simulink model "FeedBack_Linearization"  (R2021b)
settings: Solver=VariableStepAuto  StartTime=0.0  StopTime=10.0  RelTol=1e-3
undefined symbols (not defined in the file or in its folder): Kd, Kp, q_dq_init
(part 1 of 3)
settings Model: Creator=Yafei Ou  LastModifiedBy=ouyaf

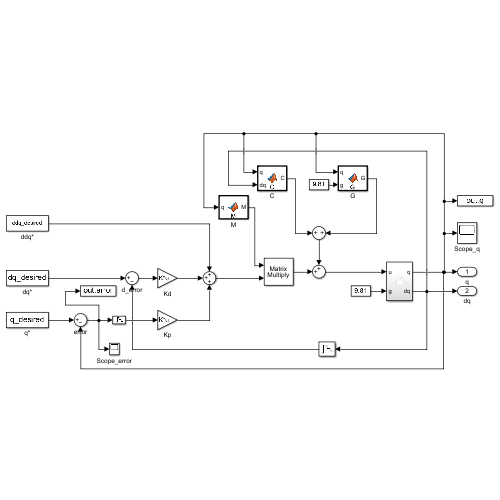
[thumbnail: Simulink's stored preview of the top-level diagram]
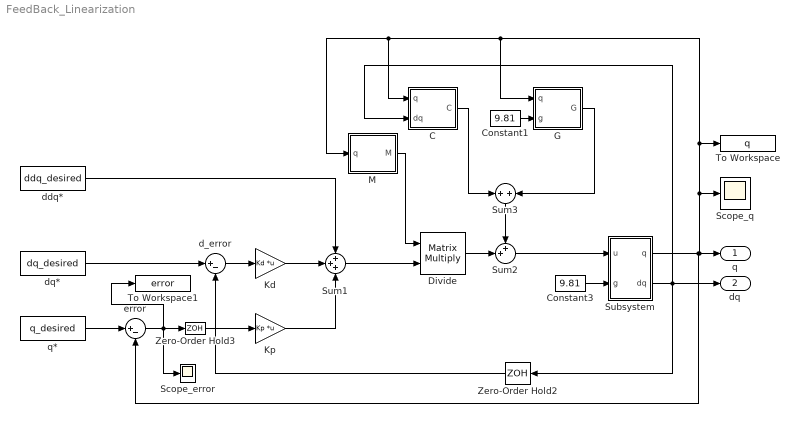
== system FeedBack_Linearization ==
  C : MATLAB Function  TreatAsAtomicUnit=on
  Constant1 : Constant  Value=9.81
  Constant3 : Constant  Value=9.81
  Divide : Product  Inputs=**  Multiplication=Matrix(*)
  G : MATLAB Function  TreatAsAtomicUnit=on
  Kd : Gain  Gain=Kd  Multiplication=Matrix(K*u)
  Kp : Gain  Gain=Kp  Multiplication=Matrix(K*u)
  M : MATLAB Function  TreatAsAtomicUnit=on
  Scope_error : Scope
  Scope_q : Scope
  Subsystem : Subsystem
  Sum1 : Sum  Inputs=+++
  Sum2 : Sum  Inputs=++|
  Sum3 : Sum  Inputs=+|+
  To Workspace : ToWorkspace  VariableName=q  SaveFormat=Timeseries  SampleTime=-1
  To Workspace1 : ToWorkspace  VariableName=error  SaveFormat=Timeseries  SampleTime=-1
  Zero-Order Hold2 : ZeroOrderHold  SampleTime=0.01
  Zero-Order Hold3 : ZeroOrderHold  SampleTime=0.01
  d_error : Sum  Inputs=|+-
  ddq* : FromWorkspace  VariableName=ddq_desired
  dq* : FromWorkspace  VariableName=dq_desired
  error : Sum  Inputs=|+-
  q* : FromWorkspace  VariableName=q_desired
  q : Outport  PortDimensions=6
  dq : Outport  Port=2
  wires:
  M/1(M) -> Divide/1
  Zero-Order Hold2/1 -> d_error/2
  C/1(C) -> Sum3/1
  Kp/1 -> Sum1/3
  Divide/1 -> Sum2/2
  Kd/1 -> Sum1/2
  dq*/1 -> d_error/1
  error/1 -> Zero-Order Hold3/1, Scope_error/1, To Workspace1/1
  Sum1/1 -> Divide/2
  Constant1/1 -> G/2(g)
  d_error/1 -> Kd/1
  q*/1 -> error/1
  Subsystem/1(q) -> q/1, Scope_q/1, To Workspace/1, G/1(q), M/1(q), C/1(q), error/2
  G/1(G) -> Sum3/2
  Sum3/1 -> Sum2/1
  ddq*/1 -> Sum1/1
  Subsystem/2(dq) -> dq/1, Zero-Order Hold2/1, C/2(dq)
  Sum2/1 -> Subsystem/1(u)
  Constant3/1 -> Subsystem/2(g)
  Zero-Order Hold3/1 -> Kp/1

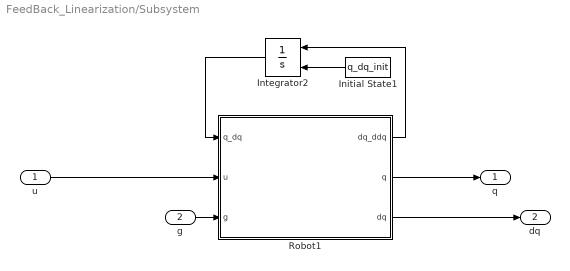
== system FeedBack_Linearization/Subsystem ==
  u : Inport
  g : Inport  Port=2
  Initial State1 : Constant  Value=q_dq_init
  Integrator2 : Integrator  InitialConditionSource=external
  Robot1 : MATLAB Function  TreatAsAtomicUnit=on
  q : Outport
  dq : Outport  Port=2
  wires:
  Integrator2/1 -> Robot1/1(q_dq)
  u/1 -> Robot1/2(u)
  Robot1/1(dq_ddq) -> Integrator2/1
  Initial State1/1 -> Integrator2/2
  Robot1/2(q) -> q/1
  Robot1/3(dq) -> dq/1
  g/1 -> Robot1/3(g)

== matlab function FeedBack_Linearization/M ==
  data: q input; M output
function M = M(q)
%M_fun
%    M = M_fun(Q1,Q2,Q3,Q4,Q5,Q6)

%    This function was generated by the Symbolic Math Toolbox version 9.0.
%    28-Mar-2022 14:36:49

q1 = q(1);
q2 = q(2);
q3 = q(3);
q4 = q(4);
q5 = q(5);
q6 = q(6);

t2 = cos(q1);
t3 = cos(q2);
t4 = cos(q4);
t5 = cos(q5);
t6 = cos(q6);
t7 = sin(q1);
t8 = sin(q2);
t9 = sin(q4);
t10 = sin(q5);
t11 = sin(q6);
t12 = q2.*2.0;
t13 = q3.^2;
t86 = q3-5.6e-3;
t120 = q3-1.56e-2;
t14 = t2.^2;
t15 = t3.^2;
t16 = t4.^2;
t17 = sin(t12);
t18 = t7.^2;
t19 = t8.^2;
t20 = t9.^2;
t21 = t2.*t4;
t22 = t3.*t5;
t23 = t2.*t9;
t24 = t4.*t7;
t25 = t3.*t10;
t26 = t5.*t8;
t27 = t7.*t9;
t28 = t8.*t10;
t29 = t3.*1.56e+2;
t33 = t8.*t9.*t11;
t38 = t3.*t4.*t6;
t49 = t3.*t4.*t11;
t50 = t3.*t6.*t9;
t62 = t3.*t9.*t11;
t63 = t6.*t8.*t9;
t68 = t2.*t8.*1.56e+2;
t71 = t7.*t8.*1.56e+2;
t76 = t3.*(7.0./1.0e+3);
t77 = q3.*t3.*1.0e+4;
t90 = t3.*t4.*t8.*t9;
t119 = q3.*t8.*(7.0./1.0e+3);
t146 = t86.^2;
t148 = q3.*t2.*t8.*1.0e+4;
t150 = q3.*t7.*t8.*1.0e+4;
t172 = q3.*t2.*t3.*-1.0e+4;
t173 = q3.*t3.*t7.*-1.0e+4;
t223 = t3.*t120;
t224 = t3.*1.79e-3;
t274 = t2.*t8.*t120;
t277 = t7.*t8.*t120;
t278 = t8.*3.2774e-3;
t309 = (t3.*t8.*t86)./1.0e+2;
t30 = t8.*t27;
t31 = t7.*t28;
t32 = t10.*t27;
t34 = t11.*t28;
t35 = t2.*t22;
t36 = t5.*t21;
t37 = t4.*t22;
t39 = t6.*t22;
t40 = t8.*t21;
t41 = t2.*t25;
t42 = t2.*t26;
t43 = t7.*t22;
t44 = t10.*t21;
t45 = t5.*t23;
t46 = t5.*t24;
t47 = t4.*t25;
t48 = t4.*t26;
t51 = t11.*t22;
t52 = t6.*t26;
t53 = t8.*t23;
t54 = t8.*t24;
t55 = t2.*t28;
t56 = t7.*t25;
t57 = t7.*t26;
t58 = t10.*t23;
t59 = t10.*t24;
t60 = t5.*t27;
t61 = t4.*t28;
t64 = t11.*t26;
t65 = t6.*t28;
t66 = t22.*9.1e+1;
t67 = t2.*t29;
t69 = t7.*t29;
t70 = t28.*9.1e+1;
t74 = -t68;
t75 = -t71;
t78 = t21.*t22;
t80 = t21.*t25;
t81 = t21.*t26;
t82 = t22.*t24;
t83 = t3.*t6.*t23;
t87 = t21.*t28;
t88 = t23.*t26;
t89 = t24.*t25;
t91 = t24.*t26;
t92 = t3.*t11.*t23;
t93 = t3.*t6.*t27;
t95 = t6.*t9.*t25;
t97 = t15.*t20;
t100 = t23.*t28;
t101 = t24.*t28;
t102 = t26.*t27;
t103 = t3.*t11.*t27;
t104 = t9.*t11.*t25;
t108 = -t50;
t109 = t27.*t28;
t112 = t22./1.0e+2;
t114 = t11.*t27.*1.0e+2;
t115 = t33.*1.0e+2;
t116 = t28./1.0e+2;
t117 = -t76;
t118 = -t77;
t123 = t6.*t21.*1.0e+2;
t130 = t11.*t21.*1.0e+2;
t131 = t6.*t24.*1.0e+2;
t132 = t49.*1.0e+2;
t133 = t50.*1.0e+2;
t139 = t9.*t25.*9.1e+1;
t141 = t11.*t23.*1.0e+2;
t142 = t11.*t24.*1.0e+2;
t147 = t2.*t77;
t149 = t7.*t77;
t232 = t90./1.0e+1;
t244 = -t224;
t272 = t2.*t223;
t275 = t7.*t223;
t283 = (t8.*t9.*t25)./1.0e+4;
t329 = t14.*t309;
t330 = t18.*t309;
t334 = t3.*t8.*t14.*t86.*(-1.0./1.0e+2);
t335 = t3.*t8.*t18.*t86.*(-1.0./1.0e+2);
t72 = -t66;
t73 = -t30;
t79 = t6.*t37;
t84 = t11.*t37;
t85 = t6.*t47;
t94 = t11.*t47;
t96 = t6.*t61;
t98 = -t37;
t99 = -t39;
t105 = t4.*t34;
t106 = -t40;
t107 = -t43;
t110 = -t60;
t111 = -t61;
t113 = t32.*9.1e+1;
t121 = t35.*9.1e+1;
t122 = t37.*9.1e+1;
t124 = t39.*1.0e+2;
t125 = t41.*9.1e+1;
t126 = t42.*9.1e+1;
t127 = t43.*9.1e+1;
t128 = t44.*9.1e+1;
t129 = t45.*9.1e+1;
t134 = t56.*9.1e+1;
t135 = t57.*9.1e+1;
t136 = t58.*9.1e+1;
t137 = t59.*9.1e+1;
t138 = t60.*9.1e+1;
t140 = t61.*9.1e+1;
t143 = t64.*1.0e+2;
t144 = t65.*1.0e+2;
t151 = t5.*t97;
t152 = -t78;
t154 = -t82;
t155 = -t83;
t157 = -t87;
t158 = -t93;
t159 = -t95;
t163 = -t102;
t166 = -t130;
t167 = -t132;
t168 = -t133;
t169 = -t109;
t171 = t32./1.0e+2;
t174 = t6.*t35.*1.0e+2;
t176 = t80.*9.1e+1;
t177 = t81.*9.1e+1;
t178 = t11.*t35.*1.0e+2;
t179 = t6.*t41.*1.0e+2;
t180 = t6.*t42.*1.0e+2;
t182 = t6.*t44.*1.0e+2;
t183 = t6.*t45.*1.0e+2;
t184 = t21.*t70;
t185 = t89.*9.1e+1;
t186 = t91.*9.1e+1;
t187 = t92.*1.0e+2;
t188 = t11.*t40.*1.0e+2;
t189 = t6.*t53.*1.0e+2;
t190 = t11.*t43.*1.0e+2;
t191 = t6.*t56.*1.0e+2;
t192 = t7.*t52.*1.0e+2;
t193 = t6.*t58.*1.0e+2;
t194 = t6.*t59.*1.0e+2;
t195 = t6.*t60.*1.0e+2;
t197 = t95.*1.0e+2;
t199 = t35./1.0e+2;
t200 = t37./1.0e+2;
t201 = t23.*t70;
t202 = t24.*t70;
t203 = t11.*t53.*1.0e+2;
t204 = t103.*1.0e+2;
t205 = t11.*t54.*1.0e+2;
t206 = t6.*t30.*1.0e+2;
t207 = t11.*t58.*1.0e+2;
t208 = t6.*t32.*1.0e+2;
t209 = t41./1.0e+2;
t210 = t42./1.0e+2;
t211 = t43./1.0e+2;
t212 = t44./1.0e+2;
t213 = t45./1.0e+2;
t214 = t27.*t70;
t215 = t11.*t30.*1.0e+2;
t216 = t11.*t32.*1.0e+2;
t217 = t56./1.0e+2;
t218 = t57./1.0e+2;
t219 = t58./1.0e+2;
t220 = t59./1.0e+2;
t221 = t60./1.0e+2;
t222 = t61./1.0e+2;
t225 = t25+t48;
t226 = t26+t47;
t227 = t23+t54;
t228 = t24+t53;
t231 = t7.*t39.*-1.0e+2;
t236 = t97./1.0e+1;
t240 = t109.*-9.1e+1;
t245 = t6.*t80.*1.0e+2;
t246 = t21.*t52.*1.0e+2;
t248 = t6.*t89.*1.0e+2;
t249 = t24.*t52.*1.0e+2;
t250 = t21.*t34.*1.0e+2;
t253 = t80./1.0e+2;
t254 = t81./1.0e+2;
t255 = t24.*t34.*1.0e+2;
t257 = t87./1.0e+2;
t258 = t89./1.0e+2;
t259 = t91./1.0e+2;
t260 = t100./1.0e+2;
t261 = t101./1.0e+2;
t262 = t109./1.0e+2;
t269 = t27.*t65.*-1.0e+2;
t284 = t42+t80;
t285 = t46+t88;
t286 = t38+t104;
t287 = t57+t89;
t288 = t59+t100;
t291 = -t283;
t333 = t45+t56+t91;
t145 = -t113;
t153 = -t79;
t156 = -t84;
t160 = -t121;
t161 = -t122;
t162 = -t124;
t164 = -t105;
t165 = -t127;
t170 = -t138;
t175 = t79.*1.0e+2;
t181 = t7.*t124;
t196 = t94.*1.0e+2;
t198 = t96.*1.0e+2;
t229 = -t174;
t233 = -t188;
t234 = -t190;
t235 = -t195;
t237 = -t200;
t238 = -t206;
t239 = -t208;
t241 = -t219;
t242 = -t221;
t243 = -t222;
t247 = t21.*t144;
t251 = t23.*t144;
t252 = t24.*t144;
t256 = t27.*t144;
t263 = t22+t111;
t264 = t28+t98;
t265 = t21+t73;
t266 = t27+t106;
t267 = t151./1.0e+1;
t268 = -t250;
t270 = -t257;
t271 = t228.^2;
t273 = -t261;
t276 = -t262;
t279 = t6.*t227;
t280 = t6.*t228;
t281 = t11.*t227;
t282 = t11.*t228;
t292 = t3.*t4.*t226;
t293 = t3.*t9.*t225;
t294 = t3.*t9.*t226;
t295 = t8.*t9.*t226;
t302 = t55+t152;
t304 = t36+t163;
t305 = t49+t159;
t306 = t31+t154;
t308 = t44+t169;
t311 = t6.*t284;
t312 = t3.*t21.*t228;
t313 = t11.*t284;
t314 = t6.*t287;
t315 = t11.*t287;
t316 = t6.*t288;
t318 = t11.*t288;
t332 = t52+t62+t85;
t339 = t41+t81+t110;
t340 = t32+t35+t157;
t341 = t33+t96+t99;
t342 = t64+t94+t108;
t343 = t58+t101+t107;
t347 = t333.^2;
t348 = t220+t260;
t349 = t227.*t228;
t363 = t228.*t285;
t374 = t139+t167+t197;
t393 = t228.*t333;
t395 = t213+t217+t259;
t409 = t218+t258+t277;
t411 = t287.*t333;
t419 = t210+t253+t274;
t496 = t129+t134+t183+t186+t191+t249;
t508 = t128+t141+t182+t205+t240+t269;
t542 = t75+t135+t150+t185+t192+t204+t248;
t543 = t74+t126+t148+t176+t180+t187+t245;
t230 = -t175;
t289 = t264.^2;
t290 = t265.^2;
t296 = t6.*t265;
t297 = t6.*t266;
t298 = -t279;
t299 = t11.*t265;
t300 = t11.*t266;
t301 = -t282;
t303 = t65+t153;
t307 = t34+t156;
t310 = t271./1.0e+1;
t317 = -t294;
t322 = -t312;
t323 = t3.*t24.*t265;
t324 = t9.*t25.*t264;
t325 = t6.*t308;
t326 = t293./1.0e+1;
t327 = t294./1.0e+1;
t328 = t11.*t308;
t336 = t312./1.0e+1;
t337 = t116+t237;
t344 = t51+t63+t164;
t346 = t332.^2;
t350 = t212+t276;
t351 = t339.^2;
t352 = t6.*t340;
t353 = t6.*t343;
t354 = t11.*t340;
t355 = t11.*t343;
t356 = t6.*t347;
t357 = t92+t311;
t358 = t103+t314;
t359 = t263.*t264;
t360 = t265.*t266;
t361 = t349./1.0e+1;
t364 = t155+t313;
t365 = t158+t315;
t367 = t3.*t23.*t340;
t368 = t9.*t22.*t342;
t369 = t3.*t27.*t343;
t373 = t228.*t302;
t375 = t143+t168+t196;
t376 = t265.*t306;
t381 = t264.*t305;
t382 = t265.*t304;
t383 = t363./1.0e+1;
t387 = (t2.*t3.*t348)./1.0e+2;
t388 = t112+t223+t243;
t401 = t209+t242+t254;
t402 = t225.*t342;
t403 = t226.*t342;
t404 = t228.*t340;
t405 = t227.*t343;
t406 = t228.*t343;
t410 = t286.*t332;
t412 = t265.*t339;
t413 = t264.*t341;
t414 = t264.*t342;
t416 = t265.*t340;
t417 = t266.*t340;
t418 = t393./1.0e+1;
t420 = t265.*t343;
t423 = t284.*t339;
t426 = t288.*t339;
t427 = t308.*t333;
t432 = (t8.*t374)./1.0e+6;
t442 = (t3.*t7.*t395)./1.0e+2;
t449 = t333.*t340;
t451 = (t3.*t7.*t409)./1.0e+2;
t454 = (t2.*t3.*t419)./1.0e+2;
t456 = t339.*t343;
t461 = t171+t199+t270+t272;
t462 = t211+t241+t273+t275;
t467 = t292.*1.0e-1;
t468 = t295.*1.0e-1;
t471 = t131+t178+t189+t216+t268;
t472 = t123+t207+t234+t238+t255;
t478 = (t2.*t3.*(t211-t219+t273+t275))./1.0e+2;
t484 = t347.*1.0e-1;
t493 = t29+t72+t115+t118+t140+t162+t198;
t503 = t114+t137+t194+t201+t233+t251;
t507 = t125+t170+t177+t179+t235+t246;
t517 = (t348.*t419)./1.0e+2;
t547 = t411.*1.0e-1;
t561 = (t3.*t7.*t496)./1.0e+6;
t567 = (t395.*t409)./1.0e+2;
t568 = (t3.*t7.*t508)./1.0e+6;
t574 = (t348.*(t211-t219+t273+t275))./1.0e+2;
t589 = (t3.*t7.*t542)./1.0e+6;
t590 = (t2.*t3.*t543)./1.0e+6;
t606 = (t419.*(t211-t219+t273+t275))./1.0e+2;
t620 = t69+t136+t165+t166+t173+t193+t202+t215+t231+t252;
t621 = t67+t142+t145+t160+t172+t184+t203+t229+t239+t247;
t639 = (t3.*t7.*(t67+t87.*9.1e+1+t142+t145-t147+t160+t203+t229+t239+t247))./1.0e+6;
t658 = (t496.*t508)./1.0e+10;
t663 = (t496.*t542)./1.0e+10;
t668 = (t508.*t542)./1.0e+10;
t699 = (t496.*(t67+t87.*9.1e+1+t142+t145-t147+t160+t203+t229+t239+t247))./1.0e+10;
t702 = (t508.*(t67+t87.*9.1e+1+t142+t145-t147+t160+t203+t229+t239+t247))./1.0e+10;
t711 = (t542.*(t67+t87.*9.1e+1+t142+t145-t147+t160+t203+t229+t239+t247))./1.0e+10;
t319 = -t297;
t320 = -t299;
t321 = t290./1.0e+1;
t331 = -t327;
t338 = -t336;
t345 = t323./1.0e+1;
t362 = t6.*t351;
t366 = (t8.*t337)./1.0e+2;
t370 = -t359;
t371 = -t360;
t377 = -t368;
t378 = -t369;
t379 = t360./1.0e+1;
t380 = t264.*t303;
t385 = -t376;
t386 = t368./1.0e+1;
t389 = t373./1.0e+1;
t391 = (t3.*t7.*t350)./1.0e+2;
t392 = (t9.*t25.*t337)./1.0e+4;
t394 = t376./1.0e+1;
t397 = t300+t316;
t398 = t281+t325;
t399 = t382./1.0e+1;
t408 = t298+t328;
t415 = t97+t271+t290;
t421 = -t406;
t422 = t70+t144+t161+t230;
t424 = -t410;
t425 = t307.*t332;
t428 = t402./1.0e+1;
t429 = t403./1.0e+1;
t430 = t404./1.0e+1;
t431 = (t8.*t388)./1.0e+2;
t433 = (t8.*t375)./1.0e+6;
t434 = t280+t354;
t435 = -t426;
t436 = t412./1.0e+1;
t437 = t420./1.0e+1;
t438 = -t432;
t440 = t301+t352;
t441 = t296+t355;
t443 = (t2.*t3.*t401)./1.0e+2;
t444 = -t442;
t446 = (t282-t352).^2;
t448 = (t9.*t25.*t388)./1.0e+4;
t450 = t332.*t344;
t453 = (t299-t353).^2;
t455 = -t451;
t457 = -t454;
t458 = t90+t322+t323;
t459 = t333.*t358;
t465 = t339.*t357;
t466 = t289.*1.0e-1;
t470 = t324.*1.0e-1;
t475 = (t3.*t7.*t461)./1.0e+2;
t481 = -t478;
t482 = (t337.*t388)./1.0e+2;
t483 = t346.*1.0e-1;
t491 = t356.*1.0e-1;
t492 = t351.*1.0e-1;
t495 = t359.*1.0e-1;
t501 = t289+t347+t351;
t505 = t367.*1.0e-1;
t506 = t369.*1.0e-1;
t509 = (t348.*t401)./1.0e+2;
t510 = (t350.*t395)./1.0e+2;
t513 = -t333.*(t282-t352);
t521 = t381.*1.0e-1;
t524 = (t2.*t3.*t471)./1.0e+6;
t525 = -t517;
M = ft_1({q3,t10,t11,t117,t119,t13,t14,t142,t145,t146,t147,t15,t151,t16,t160,t17,t18,t19,t2,t20,t203,t211,t219,t229,t232,t236,t239,t244,t247,t267,t273,t275,t278,t279,t282,t285,t291,t292,t293,t295,t297,t299,t3,t302,t304,t306,t309,t310,t313,t315,t317,t318,t319,t320,t321,t324,t326,t328,t331,t333,t334,t335,t337,t338,t339,t340,t343,t345,t346,t348,t349,t350,t352,t353,t356,t361,t362,t363,t366,t367,t370,t371,t373,t374,t375,t377,t378,t379,t380,t381,t382,t383,t385,t386,t387,t388,t389,t391,t392,t393,t394,t395,t397,t398,t399,t401,t402,t403,t404,t405,t406,t409,t410,t411,t412,t413,t414,t415,t416,t417,t418,t419,t420,t421,t422,t423,t424,t425,t426,t427,t428,t429,t430,t431,t433,t434,t435,t436,t437,t438,t441,t443,t444,t446,t448,t449,t450,t453,t455,t456,t457,t458,t459,t461,t465,t466,t467,t468,t470,t471,t472,t475,t481,t482,t483,t484,t491,t492,t493,t495,t496,t501,t503,t505,t506,t507,t508,t509,t510,t513,t521,t524,t525,t542,t543,t547,t561,t567,t568,t574,t589,t590,t606,t620,t639,t658,t663,t668,t67,t699,t7,t702,t711,t8,t83,t87,t93,t97});
end
function M = ft_1(ct)
q3 = ct{1};
t10 = ct{2};
t11 = ct{3};
t117 = ct{4};
t119 = ct{5};
t13 = ct{6};
t14 = ct{7};
t142 = ct{8};
t145 = ct{9};
t146 = ct{10};
t147 = ct{11};
t15 = ct{12};
t151 = ct{13};
t16 = ct{14};
t160 = ct{15};
t17 = ct{16};
t18 = ct{17};
t19 = ct{18};
t2 = ct{19};
t20 = ct{20};
t203 = ct{21};
t211 = ct{22};
t219 = ct{23};
t229 = ct{24};
t232 = ct{25};
t236 = ct{26};
t239 = ct{27};
t244 = ct{28};
t247 = ct{29};
t267 = ct{30};
t273 = ct{31};
t275 = ct{32};
t278 = ct{33};
t279 = ct{34};
t282 = ct{35};
t285 = ct{36};
t291 = ct{37};
t292 = ct{38};
t293 = ct{39};
t295 = ct{40};
t297 = ct{41};
t299 = ct{42};
t3 = ct{43};
t302 = ct{44};
t304 = ct{45};
t306 = ct{46};
t309 = ct{47};
t310 = ct{48};
t313 = ct{49};
t315 = ct{50};
t317 = ct{51};
t318 = ct{52};
t319 = ct{53};
t320 = ct{54};
t321 = ct{55};
t324 = ct{56};
t326 = ct{57};
t328 = ct{58};
t331 = ct{59};
t333 = ct{60};
t334 = ct{61};
t335 = ct{62};
t337 = ct{63};
t338 = ct{64};
t339 = ct{65};
t340 = ct{66};
t343 = ct{67};
t345 = ct{68};
t346 = ct{69};
t348 = ct{70};
t349 = ct{71};
t350 = ct{72};
t352 = ct{73};
t353 = ct{74};
t356 = ct{75};
t361 = ct{76};
t362 = ct{77};
t363 = ct{78};
t366 = ct{79};
t367 = ct{80};
t370 = ct{81};
t371 = ct{82};
t373 = ct{83};
t374 = ct{84};
t375 = ct{85};
t377 = ct{86};
t378 = ct{87};
t379 = ct{88};
t380 = ct{89};
t381 = ct{90};
t382 = ct{91};
t383 = ct{92};
t385 = ct{93};
t386 = ct{94};
t387 = ct{95};
t388 = ct{96};
t389 = ct{97};
t391 = ct{98};
t392 = ct{99};
t393 = ct{100};
t394 = ct{101};
t395 = ct{102};
t397 = ct{103};
t398 = ct{104};
t399 = ct{105};
t401 = ct{106};
t402 = ct{107};
t403 = ct{108};
t404 = ct{109};
t405 = ct{110};
t406 = ct{111};
t409 = ct{112};
t410 = ct{113};
t411 = ct{114};
t412 = ct{115};
t413 = ct{116};
t414 = ct{117};
t415 = ct{118};
t416 = ct{119};
t417 = ct{120};
t418 = ct{121};
t419 = ct{122};
t420 = ct{123};
t421 = ct{124};
t422 = ct{125};
t423 = ct{126};
t424 = ct{127};
t425 = ct{128};
t426 = ct{129};
t427 = ct{130};
t428 = ct{131};
t429 = ct{132};
t430 = ct{133};
t431 = ct{134};
t433 = ct{135};
t434 = ct{136};
t435 = ct{137};
t436 = ct{138};
t437 = ct{139};
t438 = ct{140};
t441 = ct{141};
t443 = ct{142};
t444 = ct{143};
t446 = ct{144};
t448 = ct{145};
t449 = ct{146};
t450 = ct{147};
t453 = ct{148};
t455 = ct{149};
t456 = ct{150};
t457 = ct{151};
t458 = ct{152};
t459 = ct{153};
t461 = ct{154};
t465 = ct{155};
t466 = ct{156};
t467 = ct{157};
t468 = ct{158};
t470 = ct{159};
t471 = ct{160};
t472 = ct{161};
t475 = ct{162};
t481 = ct{163};
t482 = ct{164};
t483 = ct{165};
t484 = ct{166};
t491 = ct{167};
t492 = ct{168};
t493 = ct{169};
t495 = ct{170};
t496 = ct{171};
t501 = ct{172};
t503 = ct{173};
t505 = ct{174};
t506 = ct{175};
t507 = ct{176};
t508 = ct{177};
t509 = ct{178};
t510 = ct{179};
t513 = ct{180};
t521 = ct{181};
t524 = ct{182};
t525 = ct{183};
t542 = ct{184};
t543 = ct{185};
t547 = ct{186};
t561 = ct{187};
t567 = ct{188};
t568 = ct{189};
t574 = ct{190};
t589 = ct{191};
t590 = ct{192};
t606 = ct{193};
t620 = ct{194};
t639 = ct{195};
t658 = ct{196};
t663 = ct{197};
t668 = ct{198};
t67 = ct{199};
t699 = ct{200};
t7 = ct{201};
t702 = ct{202};
t711 = ct{203};
t8 = ct{204};
t83 = ct{205};
t87 = ct{206};
t93 = ct{207};
t97 = ct{208};
t526 = (t350.*t409)./1.0e+2;
t528 = (t3.*t7.*t472)./1.0e+6;
t529 = -t11.*t339.*(t282-t352);
t530 = -t11.*t333.*(t299-t353);
t531 = -t339.*(t299-t353);
t533 = t151+t363+t382;
t534 = t11.*t333.*(t299-t353);
t537 = t405.*1.0e-1;
t538 = t406.*1.0e-1;
t539 = t393+t412;
t540 = (t83-t313).*(t282-t352);
t541 = (t8.*t493)./1.0e+6;
t546 = t410.*1.0e-1;
t548 = t413.*1.0e-1;
t549 = t414.*1.0e-1;
t550 = (t374.*t375)./1.0e+10;
t551 = t416.*1.0e-1;
t552 = t417.*1.0e-1;
t554 = (t93-t315).*(t299-t353);
t556 = t423.*1.0e-1;
t558 = t426.*1.0e-1;
t559 = t427.*1.0e-1;
t563 = -t561;
t564 = (t2.*t3.*t503)./1.0e+6;
t566 = (t2.*t3.*t507)./1.0e+6;
t570 = (t401.*t419)./1.0e+2;
t571 = -t568;
t573 = (t350.*t461)./1.0e+2;
t576 = (t297-t318).*(t282-t352);
t578 = -t574;
t581 = t449.*1.0e-1;
t585 = (t279-t328).*(t299-t353);
t587 = t456.*1.0e-1;
t591 = -t589;
t593 = -t590;
t598 = (t395.*t461)./1.0e+2;
t601 = t292+t405+t417;
t602 = (t401.*(t211-t219+t273+t275))./1.0e+2;
t603 = (t409.*t461)./1.0e+2;
t604 = t317+t404+t420;
t609 = t449+t456;
t614 = t333.*(t282-t352).*(-1.0e-1);
t622 = t11.*t339.*(t282-t352).*(-1.0e-1);
t623 = (t374.*t493)./1.0e+10;
t624 = (t375.*t493)./1.0e+10;
t626 = t339.*(t299-t353).*(-1.0e-1);
t638 = (t2.*t3.*t620)./1.0e+6;
t641 = -t639;
t646 = (t472.*t496)./1.0e+10;
t647 = (t471.*t503)./1.0e+10;
t648 = (t471.*t507)./1.0e+10;
t651 = (t472.*t508)./1.0e+10;
t656 = (t471.*t543)./1.0e+10;
t657 = (t472.*t542)./1.0e+10;
t659 = (t503.*t507)./1.0e+10;
t664 = (t503.*t543)./1.0e+10;
t669 = (t507.*t543)./1.0e+10;
t682 = (t471.*t620)./1.0e+10;
t684 = (t472.*(t67+t87.*9.1e+1+t142+t145-t147+t160+t203+t229+t239+t247))./1.0e+10;
t698 = (t503.*t620)./1.0e+10;
t701 = (t507.*t620)./1.0e+10;
t709 = (t543.*t620)./1.0e+10;
t372 = -t366;
t384 = -t379;
t390 = -t386;
t396 = -t391;
t400 = -t394;
t407 = t318+t319;
t439 = -t433;
t445 = t320+t353;
t447 = -t443;
t452 = -t448;
t460 = (t8.*t422)./1.0e+6;
t464 = t236+t310+t321;
t469 = t349+t371;
t473 = t333.*t398;
t474 = t285.*t434;
t476 = t232+t338+t345;
t479 = t302.*t434;
t480 = t339.*t397;
t485 = t306.*t441;
t486 = -t482;
t490 = t304.*t441;
t497 = t362.*1.0e-1;
t499 = t333.*t434;
t502 = -t495;
t511 = t339.*t434;
t512 = t340.*t434;
t514 = t333.*t441;
t515 = -t506;
t516 = -t509;
t518 = t380.*1.0e-1;
t519 = t339.*t441;
t523 = t343.*t441;
t527 = -t524;
t544 = -t538;
t545 = -t541;
t553 = -t540;
t555 = -t546;
t557 = t425.*1.0e-1;
t560 = t416+t421;
t562 = -t558;
t565 = t295+t367+t378;
t569 = -t566;
t572 = t418+t436;
t575 = t293+t373+t385;
t577 = -t573;
t579 = t267+t383+t399;
t580 = t446.*1.0e-1;
t582 = t450.*1.0e-1;
t583 = (t374.*t422)./1.0e+10;
t584 = (t375.*t422)./1.0e+10;
t586 = t453.*1.0e-1;
t588 = t459.*1.0e-1;
t592 = t356+t362+t380;
t594 = -t434.*(t299-t353);
t595 = -t441.*(t282-t352);
t596 = t465.*1.0e-1;
t597 = t441.*(t282-t352);
t600 = -t598;
t607 = -t603;
t612 = t324+t427+t435;
t617 = t331+t430+t437;
t625 = t534.*(-1.0e-1);
t627 = t534.*1.0e-1;
t628 = t370+t411+t423;
t629 = t540.*1.0e-1;
t632 = t554.*1.0e-1;
t634 = (t422.*t493)./1.0e+10;
t635 = t346+t446+t453;
t637 = t576.*1.0e-1;
t640 = t585.*1.0e-1;
t642 = t434.*(t299-t353).*(-1.0e-1);
t649 = -t646;
t650 = -t647;
t652 = t513+t531;
t653 = -t651;
t655 = t413+t459+t465;
t660 = -t657;
t661 = -t659;
t665 = -t664;
t678 = t581+t587;
t683 = -t682;
t685 = t466+t484+t492;
t686 = -t684;
t697 = t425+t529+t534;
t703 = -t701;
t710 = -t709;
t714 = t467+t537+t552;
t715 = t424+t576+t585;
t716 = t614+t626;
t790 = t117+t475+t481+t638+t641;
t463 = -t460;
t477 = -t473;
t487 = -t479;
t488 = t474./1.0e+1;
t489 = t361+t384;
t494 = t479./1.0e+1;
t500 = t485./1.0e+1;
t504 = t490./1.0e+1;
t520 = t499./1.0e+1;
t522 = -t514;
t532 = t512./1.0e+1;
t535 = t519./1.0e+1;
t536 = t523./1.0e+1;
t599 = t326+t389+t400;
t605 = t473.*1.0e-1;
t610 = t480.*1.0e-1;
t611 = (t415.*t476)./2.0;
t613 = t511.*1.0e-1;
t615 = t514.*1.0e-1;
t618 = (t458.*t464)./2.0;
t630 = (t464.*t469)./2.0;
t631 = -t629;
t636 = (t469.*t476)./2.0;
t643 = t597.*(-1.0e-1);
t644 = t597.*1.0e-1;
t645 = t499+t519;
t662 = t544+t551;
t667 = t377+t474+t490;
t670 = (t533.*t572)./2.0;
t671 = (t539.*t579)./2.0;
t675 = (t572.*t575)./2.0;
t676 = (t575.*t579)./2.0;
t680 = t403+t512+t523;
t687 = (t533.*t617)./2.0;
t688 = (t572.*t604)./2.0;
t690 = (t579.*t604)./2.0;
t692 = t594+t597;
t694 = (t539.*t617)./2.0;
t700 = t439+t527+t528;
t704 = t468+t505+t515;
t705 = (t575.*t617)./2.0;
t712 = t491+t497+t518;
t713 = t450+t553+t554;
t717 = t470+t559+t562;
t718 = t502+t547+t556;
t719 = t483+t580+t586;
t721 = (t501.*t678)./2.0;
t725 = t548+t588+t596;
t729 = (t612.*t678)./2.0;
t731 = (t609.*t685)./2.0;
t734 = (t628.*t678)./2.0;
t735 = t714.*(t406-t416).*(-1.0./2.0);
t739 = (t714.*(t406-t416))./2.0;
t741 = (t565.*t714)./2.0;
t742 = (t612.*t685)./2.0;
t745 = t291+t387+t396+t438+t564+t571;
t746 = (t628.*t685)./2.0;
t747 = t557+t622+t627;
t750 = t592.*(t333.*(t282-t352).*1.0e-1+t339.*(t299-t353).*1.0e-1).*(-1.0./2.0);
t751 = (t592.*(t333.*(t282-t352).*1.0e-1+t339.*(t299-t353).*1.0e-1))./2.0;
t759 = t555+t637+t640;
t787 = t655.*(t333.*(t282-t352).*1.0e-1+t339.*(t299-t353).*1.0e-1).*(-1.0./2.0);
t788 = (t655.*(t333.*(t282-t352).*1.0e-1+t339.*(t299-t353).*1.0e-1))./2.0;
t825 = t309+t334+t335+t431+t455+t457+t545+t591+t593-1.05e-2;
t498 = -t494;
t608 = -t605;
t616 = (t415.*t489)./2.0;
t619 = -t615;
t633 = (t458.*t489)./2.0;
t654 = t520+t535;
t666 = t381+t477+t480;
t672 = t402+t485+t487;
t673 = t390+t488+t504;
t674 = (t533.*t599)./2.0;
t677 = (t539.*t599)./2.0;
t681 = t414+t511+t522;
t689 = -t687;
t691 = -t688;
t693 = -t690;
t695 = -t694;
t696 = t429+t532+t536;
t706 = (t599.*t604)./2.0;
t707 = -t705;
t720 = (t565.*t662)./2.0;
t722 = -t721;
t723 = (t601.*t662)./2.0;
t726 = t642+t644;
t728 = t704.*(t406-t416).*(-1.0./2.0);
t730 = -t729;
t732 = -t731;
t733 = (t501.*t717)./2.0;
t736 = -t734;
t738 = (t601.*t704)./2.0;
t743 = -t741;
t744 = (t501.*t718)./2.0;
t754 = t582+t631+t632;
t757 = (t609.*t717)./2.0;
t760 = (t609.*t718)./2.0;
t766 = (t612.*t718)./2.0;
t767 = (t628.*t717)./2.0;
t772 = t372+t444+t447+t463+t563+t569;
t773 = t712.*(t333.*(t282-t352)+t339.*(t299-t353)).*(-1.0./2.0);
t775 = (t712.*(t333.*(t282-t352)+t339.*(t299-t353)))./2.0;
t779 = (t655.*t712)./2.0;
t780 = (t592.*t725)./2.0;
t797 = t725.*(t333.*(t282-t352)+t339.*(t299-t353)).*(-1.0./2.0);
t798 = (t725.*(t333.*(t282-t352)+t339.*(t299-t353)))./2.0;
t804 = (t635.*t747)./2.0;
t805 = (t692.*t719)./2.0;
t808 = (t697.*t719)./2.0;
t815 = (t713.*t719)./2.0;
t816 = (t635.*t759)./2.0;
t820 = (t715.*t719)./2.0;
t828 = (t692.*t747)./2.0;
t832 = (t713.*t747)./2.0;
t835 = (t692.*t759)./2.0;
t837 = (t697.*t759)./2.0;
t838 = (t715.*t747)./2.0;
t842 = (t713.*t759)./2.0;
t679 = t428+t498+t500;
t708 = -t706;
t724 = -t723;
t727 = t521+t608+t610;
t737 = t549+t613+t619;
t740 = -t738;
t748 = (t654.*t667)./2.0;
t749 = (t645.*t673)./2.0;
t752 = (t654.*t672)./2.0;
t758 = -t757;
t761 = (t654.*t680)./2.0;
t762 = -t760;
t764 = (t645.*t696)./2.0;
t768 = (t672.*t673)./2.0;
t774 = (t673.*t680)./2.0;
t777 = (t667.*t696)./2.0;
t782 = (t672.*t696)./2.0;
t785 = (t666.*t712)./2.0;
t789 = t666.*(t333.*(t282-t352).*1.0e-1+t339.*(t299-t353).*1.0e-1).*(-1.0./2.0);
t791 = (t635.*t726)./2.0;
t794 = (t681.*t712)./2.0;
t795 = t681.*(t333.*(t282-t352).*1.0e-1+t339.*(t299-t353).*1.0e-1).*(-1.0./2.0);
t796 = (t681.*(t333.*(t282-t352).*1.0e-1+t339.*(t299-t353).*1.0e-1))./2.0;
t802 = (t666.*t725)./2.0;
t806 = -t804;
t807 = -t805;
t809 = -t808;
t813 = (t635.*t754)./2.0;
t814 = (t681.*t725)./2.0;
t817 = (t697.*t726)./2.0;
t823 = (t713.*t726)./2.0;
t826 = (t715.*t726)./2.0;
t829 = (t692.*t754)./2.0;
t831 = (t697.*t754)./2.0;
t834 = -t832;
t836 = -t835;
t839 = -t837;
t840 = -t838;
t841 = (t715.*t754)./2.0;
t753 = -t752;
t755 = (t645.*t679)./2.0;
t763 = -t761;
t765 = -t764;
t769 = (t667.*t679)./2.0;
t770 = -t768;
t776 = -t774;
t778 = -t777;
t781 = (t679.*t680)./2.0;
t783 = (t592.*t727)./2.0;
t786 = -t785;
t792 = -t791;
t793 = (t592.*t737)./2.0;
t799 = t727.*(t333.*(t282-t352)+t339.*(t299-t353)).*(-1.0./2.0);
t800 = (t655.*t727)./2.0;
t803 = -t802;
t810 = t737.*(t333.*(t282-t352)+t339.*(t299-t353)).*(-1.0./2.0);
t811 = (t737.*(t333.*(t282-t352)+t339.*(t299-t353)))./2.0;
t812 = (t655.*t737)./2.0;
t818 = (t666.*t737)./2.0;
t819 = (t681.*t727)./2.0;
t824 = -t823;
t827 = -t826;
t830 = -t829;
t833 = -t831;
t756 = -t755;
t771 = -t769;
t784 = -t783;
t801 = -t800;
t821 = -t818;
t822 = -t819;
t843 = t584+t648+t649+t793+t794+t806+t809;
t844 = t683+t686+t792+t796+t807+t811;
t846 = t624+t656+t660+t812+t813+t814+t815;
t847 = t600+t602+t691+t695+t699+t703+t722+t732+t751+t763+t765+t775+t817+t828;
t849 = t486+t567+t570+t634+t663+t669+t707+t708+t744+t746+t779+t780+t781+t782+t833+t834;
t850 = t577+t578+t616+t630+t670+t671+t698+t702+t724+t730+t739+t748+t749+t758+t789+t799+t827+t836;
t845 = t550+t650+t653+t816+t820+t821+t822;
t848 = t392+t510+t516+t583+t658+t661+t689+t693+t733+t742+t776+t778+t784+t786+t839+t840;
t851 = t119+t244+t278+t606+t607+t633+t636+t675+t677+t710+t711+t720+t728+t736+t753+t756+t762+t788+t798+t824+t830;
t852 = t452+t525+t526+t611+t618+t623+t665+t668+t674+t676+t740+t743+t766+t767+t770+t771+t801+t803+t841+t842;
et1 = t15.*(-8.9756331066e+1)+t17.*5.5839e-3+t97.*1.0e-1+(t67+t87.*9.1e+1+t142+t145-t147+t160+t203+t229+t239+t247).^2./1.0e+10;
et2 = (t333.*(t282-t352)+t339.*(t299-t353)).*(t333.*(t282-t352).*1.0e-1+t339.*(t299-t353).*1.0e-1)-q3.*t15.*3.7226e-1-q3.*t17.*1.05e-2+t3.*t8.*(7.0./2.5e+2)+t13.*t15.*(7.0./2.0e+1)+t15.*t16.*1.0e-1;
et3 = t469.*t489+t539.*t572+t609.*t678+t645.*t654+t692.*t726-t662.*(t406-t416)+t461.^2./1.0e+2+t620.^2./1.0e+10+(t211-t219+t273+t275).^2./1.0e+2+(t14.*t15.*t146)./1.0e+2+(t15.*t18.*t146)./1.0e+2+9.0206055e+1;
et4 = q3.*(-3.7226e-1)+t13.*(7.0./2.0e+1)+t16.*1.0e-1+t20.*1.0e-1+(t15.*t146)./1.0e+2+t458.*t476+t575.*t599+t565.*t704+t628.*t718+t672.*t679+t655.*t725+t713.*t754+t388.^2./1.0e+2+t409.^2./1.0e+2+t419.^2./1.0e+2+t493.^2./1.0e+10+t542.^2./1.0e+10;
et5 = t543.^2./1.0e+10+(t14.*t19.*t146)./1.0e+2+(t18.*t19.*t146)./1.0e+2+9.0252298934e+1;
mt1 = [et1+et2+et3,t851,t790,t850,t847,t844,t851,et4+et5,t825,t852,t849,t846,t790,t825,t19.*(3.0./1.0e+2)+t14.*t15.*(3.0./1.0e+2)+t15.*t18.*(3.0./1.0e+2)+7.0./2.0e+1,t745,t772,t700,t850,t852,t745,t415.*t464+t533.*t579+t601.*t714+t612.*t717+t667.*t673+t666.*t727+t715.*t759+(t10.^2.*t97)./1.0e+6+t348.^2./1.0e+2+t350.^2./1.0e+2+t374.^2./1.0e+10+t503.^2./1.0e+10+t508.^2./1.0e+10,t848,t845,t847,t849,t772,t848];
mt2 = [t501.*t685+t604.*t617+t592.*t712+t680.*t696+t697.*t747+t337.^2./1.0e+2+t395.^2./1.0e+2+t401.^2./1.0e+2+t422.^2./1.0e+10+t496.^2./1.0e+10+t507.^2./1.0e+10,t843,t844,t846,t700,t845,t843,t635.*t719+t681.*t737+t375.^2./1.0e+10+t471.^2./1.0e+10+t472.^2./1.0e+10];
M = reshape([mt1,mt2],6,6);
end
